simulink model "ex5"  (R2015a)
settings: Solver=ode3  StartTime=0.0  StopTime=10.0  FixedStep=0.1  RelTol=1e-3
undefined symbols (not defined in the file): g, l
libraries: simulink x1
settings Model: Creator=fschalle  LastModifiedBy=fschalle

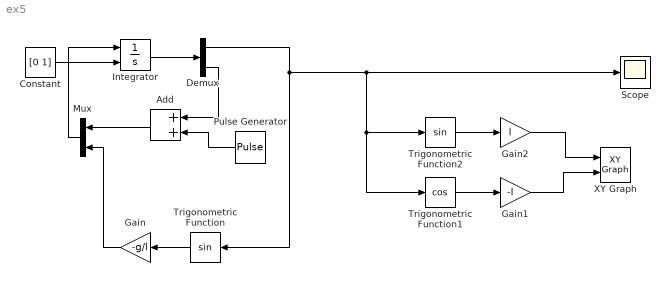
== system ex5 ==
  Add : Sum
  Constant : Constant  Value=[0 1]
  Demux : Demux  Outputs=2
  Gain : Gain  Gain=-g/l
  Gain1 : Gain  Gain=-l
  Gain2 : Gain  Gain=l
  Integrator : Integrator  InitialConditionSource=external
  Mux : Mux  Inputs=2
  Pulse Generator : DiscretePulseGenerator  PulseType=Time based  Period=0.2  PulseWidth=50
  Scope : Scope
  Trigonometric Function : Trigonometry
  Trigonometric Function1 : Trigonometry  Operator=cos
  Trigonometric Function2 : Trigonometry
  XY Graph : simulink/Sinks/XY Graph  xmin=-5  xmax=5  ymin=-5  ymax=5  st=-1
  wires:
  Constant/1 -> Integrator/2
  Integrator/1 -> Demux/1
  Gain/1 -> Mux/2
  Mux/1 -> Integrator/1
  Trigonometric Function/1 -> Gain/1
  Trigonometric Function1/1 -> Gain1/1
  Trigonometric Function2/1 -> Gain2/1
  Gain1/1 -> XY Graph/2
  Gain2/1 -> XY Graph/1
  Demux/1 -> Trigonometric Function/1, Trigonometric Function1/1, Trigonometric Function2/1, Scope/1
  Add/1 -> Mux/1
  Pulse Generator/1 -> Add/2
  Demux/2 -> Add/1
